simulink subsystem "Rocket_Motor"  (R2020b)
settings: Solver=VariableStepAuto  StartTime=0.0  StopTime=10.0  RelTol=1e-3
libraries: fl_lib x15, nesl_utility x8
settings Model: Creator=Edward  LastModifiedBy=Edward

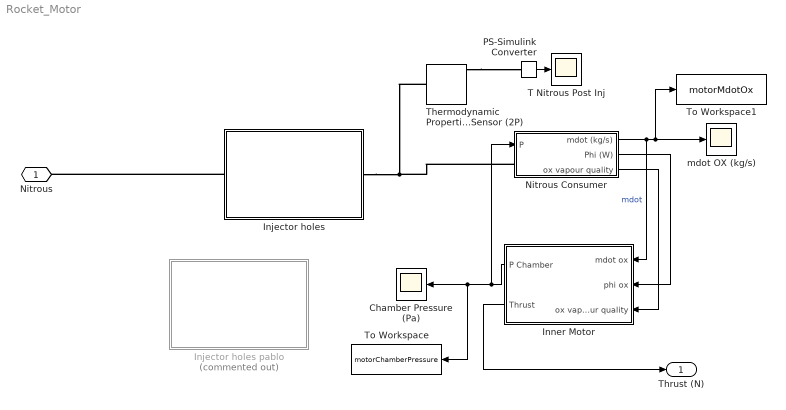
== system Rocket_Motor ==
  Chamber Pressure (Pa) : Scope
  Injector holes : Subsystem  ReferencedSubsystem=Injector
  Injector holes pablo : Subsystem  Commented=on
  Inner Motor : Subsystem
      mask Display: image('$imagefile'); % Use "Edit Image" on toolstrip to change.
  Nitrous Consumer : Subsystem
  PS-Simulink Converter : nesl_utility/PS-Simulink Converter  PhysicalDomain=network_engine_domain  SubClassName=ps_output  LeftPortType=input  RightPortType=output  PseudoPeriodic=off  Frequencies=[]  Unit=inherit  AffineConversion=off
  T Nitrous Post Inj : Scope
  Thermodynamic Properties Sensor (2P) : fl_lib/Two-Phase Fluid/Sensors/Thermodynamic Properties Sensor (2P)
      settings: SourceProductBaseCode=SS  InternalSimscapePortConfiguration="{\"Bottom\":[],\"Left\":[{\"id\":\"A\",\"label\":\"A\",\"type\":\"foundation.two_phase_fluid.two_phase_fluid\"}],\"Right\":[{\"id\":\"T\",\"label\":\"T\",\"type\":\"output\"},{\"id\":\"H\",\"label\":\"h\",\"type\":\"output\"},{\"id\":\"V\",\"label\":\"v\",\"type\":\"output\"},{\"id\":\"S\",\"label\":\"s\",\"type\":\"output\"}],\"Top\":[]}"
  To Workspace : ToWorkspace  VariableName=motorChamberPressure  SaveFormat=Timeseries  SampleTime=-1
  To Workspace1 : ToWorkspace  VariableName=motorMdotOx  SaveFormat=Timeseries  SampleTime=-1
  mdot OX (kg/s) : Scope
  Nitrous : PMIOPort  Side=Left
  Thrust (N) : Outport
  wires:
  Nitrous Consumer/1(mdot (kg/s)) -> mdot OX (kg/s)/1, To Workspace1/1, Inner Motor/1(mdot ox)  "mdot"
  Inner Motor/1(P Chamber) -> To Workspace/1, Chamber Pressure (Pa)/1, Nitrous Consumer/1(P)
  Nitrous Consumer/2(Phi (W)) -> Inner Motor/2(phi ox)
  Inner Motor/2(Thrust) -> Thrust (N)/1
  Nitrous Consumer/3(ox vapour quality) -> Inner Motor/3(ox vapour quality)
  PS-Simulink Converter/1 -> T Nitrous Post Inj/1
  connections:
  Nitrous Consumer/LConn1 -- Thermodynamic Properties Sensor (2P)/LConn1 -- Injector holes/RConn1
  Injector holes/LConn1 -- Nitrous/RConn1
  Thermodynamic Properties Sensor (2P)/RConn1 -- PS-Simulink Converter/LConn1

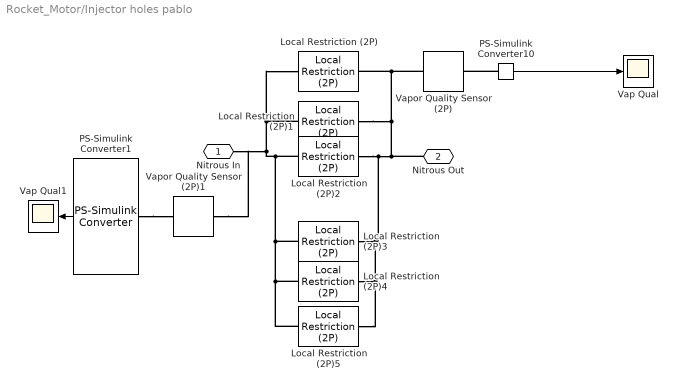
== system Rocket_Motor/Injector holes pablo ==
  Local Restriction (2P) : fl_lib/Two-Phase Fluid/Elements/Local Restriction (2P)  restriction_area=9.50e-7 m^2  area=sim.preInjectorPipe.crossSection m^2  Cd=0.64  B_lam=0.999
      settings: SourceProductBaseCode=SS  InternalSimscapePortConfiguration="{\"Bottom\":[],\"Left\":[{\"id\":\"A\",\"label\":\"A\",\"type\":\"foundation.two_phase_fluid.two_phase_fluid\"}],\"Right\":[{\"id\":\"B\",\"label\":\"B\",\"type\":\"foundation.two_phase_fluid.two_phase_fluid\"}],\"Top\":[]}"
  Local Restriction (2P)1 : fl_lib/Two-Phase Fluid/Elements/Local Restriction (2P)  restriction_area=9.50e-7 m^2  area=sim.preInjectorPipe.crossSection m^2  Cd=0.64  B_lam=0.999
      settings: SourceProductBaseCode=SS  InternalSimscapePortConfiguration="{\"Bottom\":[],\"Left\":[{\"id\":\"A\",\"label\":\"A\",\"type\":\"foundation.two_phase_fluid.two_phase_fluid\"}],\"Right\":[{\"id\":\"B\",\"label\":\"B\",\"type\":\"foundation.two_phase_fluid.two_phase_fluid\"}],\"Top\":[]}"
  Local Restriction (2P)2 : fl_lib/Two-Phase Fluid/Elements/Local Restriction (2P)  restriction_area=9.50e-7 m^2  area=sim.preInjectorPipe.crossSection m^2  Cd=0.64  B_lam=0.999
      settings: SourceProductBaseCode=SS  InternalSimscapePortConfiguration="{\"Bottom\":[],\"Left\":[{\"id\":\"A\",\"label\":\"A\",\"type\":\"foundation.two_phase_fluid.two_phase_fluid\"}],\"Right\":[{\"id\":\"B\",\"label\":\"B\",\"type\":\"foundation.two_phase_fluid.two_phase_fluid\"}],\"Top\":[]}"
  Local Restriction (2P)3 : fl_lib/Two-Phase Fluid/Elements/Local Restriction (2P)  restriction_area=4.07e-7 m^2  area=sim.preInjectorPipe.crossSection m^2  Cd=0.64  B_lam=0.999
      settings: SourceProductBaseCode=SS  InternalSimscapePortConfiguration="{\"Bottom\":[],\"Left\":[{\"id\":\"A\",\"label\":\"A\",\"type\":\"foundation.two_phase_fluid.two_phase_fluid\"}],\"Right\":[{\"id\":\"B\",\"label\":\"B\",\"type\":\"foundation.two_phase_fluid.two_phase_fluid\"}],\"Top\":[]}"
  Local Restriction (2P)4 : fl_lib/Two-Phase Fluid/Elements/Local Restriction (2P)  restriction_area=4.07e-7 m^2  area=sim.preInjectorPipe.crossSection m^2  Cd=0.64  B_lam=0.999
      settings: SourceProductBaseCode=SS  InternalSimscapePortConfiguration="{\"Bottom\":[],\"Left\":[{\"id\":\"A\",\"label\":\"A\",\"type\":\"foundation.two_phase_fluid.two_phase_fluid\"}],\"Right\":[{\"id\":\"B\",\"label\":\"B\",\"type\":\"foundation.two_phase_fluid.two_phase_fluid\"}],\"Top\":[]}"
  Local Restriction (2P)5 : fl_lib/Two-Phase Fluid/Elements/Local Restriction (2P)  restriction_area=4.07e-7 m^2  area=sim.preInjectorPipe.crossSection m^2  Cd=0.64  B_lam=0.999
      settings: SourceProductBaseCode=SS  InternalSimscapePortConfiguration="{\"Bottom\":[],\"Left\":[{\"id\":\"A\",\"label\":\"A\",\"type\":\"foundation.two_phase_fluid.two_phase_fluid\"}],\"Right\":[{\"id\":\"B\",\"label\":\"B\",\"type\":\"foundation.two_phase_fluid.two_phase_fluid\"}],\"Top\":[]}"
  PS-Simulink Converter1 : nesl_utility/PS-Simulink Converter  PhysicalDomain=network_engine_domain  SubClassName=ps_output  LeftPortType=input  RightPortType=output  PseudoPeriodic=off  Frequencies=[]  Unit=inherit  AffineConversion=off
  PS-Simulink Converter10 : nesl_utility/PS-Simulink Converter  PhysicalDomain=network_engine_domain  SubClassName=ps_output  LeftPortType=input  RightPortType=output  PseudoPeriodic=off  Frequencies=[]  Unit=inherit  AffineConversion=off
  Vap Qual : Scope
  Vap Qual1 : Scope
  Vapor Quality Sensor (2P) : fl_lib/Two-Phase Fluid/Sensors/Vapor Quality Sensor (2P)  vapor_fraction_spec=foundation.enum.vapor_fraction_spec.quality
      settings: SourceProductBaseCode=SS  InternalSimscapePortConfiguration="{\"Bottom\":[],\"Left\":[{\"id\":\"A\",\"label\":\"A\",\"type\":\"foundation.two_phase_fluid.two_phase_fluid\"}],\"Right\":[{\"id\":\"X\",\"label\":\"X\",\"type\":\"output\"}],\"Top\":[]}"
  Vapor Quality Sensor (2P)1 : fl_lib/Two-Phase Fluid/Sensors/Vapor Quality Sensor (2P)  vapor_fraction_spec=foundation.enum.vapor_fraction_spec.quality
      settings: SourceProductBaseCode=SS  InternalSimscapePortConfiguration="{\"Bottom\":[],\"Left\":[{\"id\":\"A\",\"label\":\"A\",\"type\":\"foundation.two_phase_fluid.two_phase_fluid\"}],\"Right\":[{\"id\":\"X\",\"label\":\"X\",\"type\":\"output\"}],\"Top\":[]}"
  Nitrous In : PMIOPort  Side=Left
  Nitrous Out : PMIOPort  Port=2  Side=Right
  wires:
  PS-Simulink Converter1/1 -> Vap Qual1/1
  PS-Simulink Converter10/1 -> Vap Qual/1
  connections:
  PS-Simulink Converter1/LConn1 -- Vapor Quality Sensor (2P)1/RConn1
  PS-Simulink Converter10/LConn1 -- Vapor Quality Sensor (2P)/RConn1
  Local Restriction (2P)4/LConn1 -- Local Restriction (2P)5/LConn1 -- Local Restriction (2P)3/LConn1 -- Local Restriction (2P)2/LConn1 -- Vapor Quality Sensor (2P)1/LConn1 -- Nitrous In/RConn1 -- Local Restriction (2P)/LConn1 -- Local Restriction (2P)1/LConn1
  Local Restriction (2P)5/RConn1 -- Local Restriction (2P)4/RConn1 -- Local Restriction (2P)3/RConn1 -- Local Restriction (2P)2/RConn1 -- Local Restriction (2P)/RConn1 -- Vapor Quality Sensor (2P)/LConn1 -- Local Restriction (2P)1/RConn1 -- Nitrous Out/RConn1

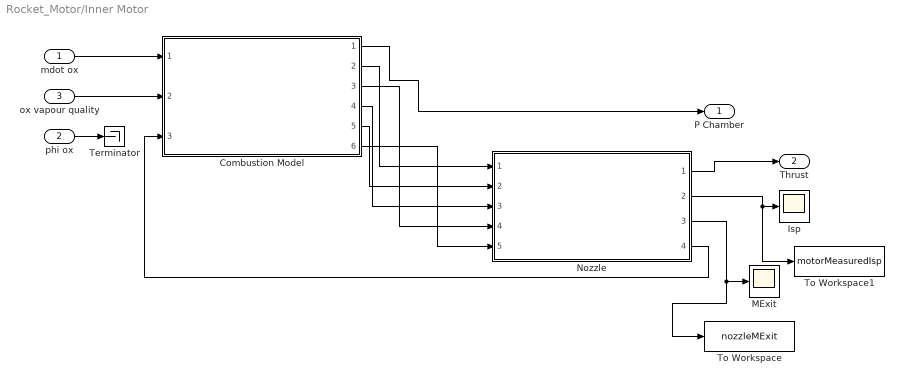
== system Rocket_Motor/Inner Motor ==
  mdot ox : Inport
  phi ox : Inport  Port=2
  ox vapour quality : Inport  Port=3
  Combustion Model : Subsystem  ReferencedSubsystem=Combustion_Model
  Isp : Scope
  MExit : Scope
  Nozzle : Subsystem  ReferencedSubsystem=Nozzle
  Terminator : Terminator
  To Workspace : ToWorkspace  VariableName=nozzleMExit  SaveFormat=Timeseries  SampleTime=-1
  To Workspace1 : ToWorkspace  VariableName=motorMeasuredIsp  SaveFormat=Timeseries  SampleTime=-1
  P Chamber : Outport
  Thrust : Outport  Port=2
  wires:
  Combustion Model/6 -> Nozzle/5
  Nozzle/4 -> Combustion Model/3
  ox vapour quality/1 -> Combustion Model/2
  Combustion Model/3 -> Nozzle/4
  phi ox/1 -> Terminator/1
  Nozzle/3 -> MExit/1, To Workspace/1
  Nozzle/2 -> Isp/1, To Workspace1/1
  Nozzle/1 -> Thrust/1
  Combustion Model/4 -> Nozzle/3
  Combustion Model/5 -> Nozzle/2
  Combustion Model/2 -> Nozzle/1
  Combustion Model/1 -> P Chamber/1
  mdot ox/1 -> Combustion Model/1

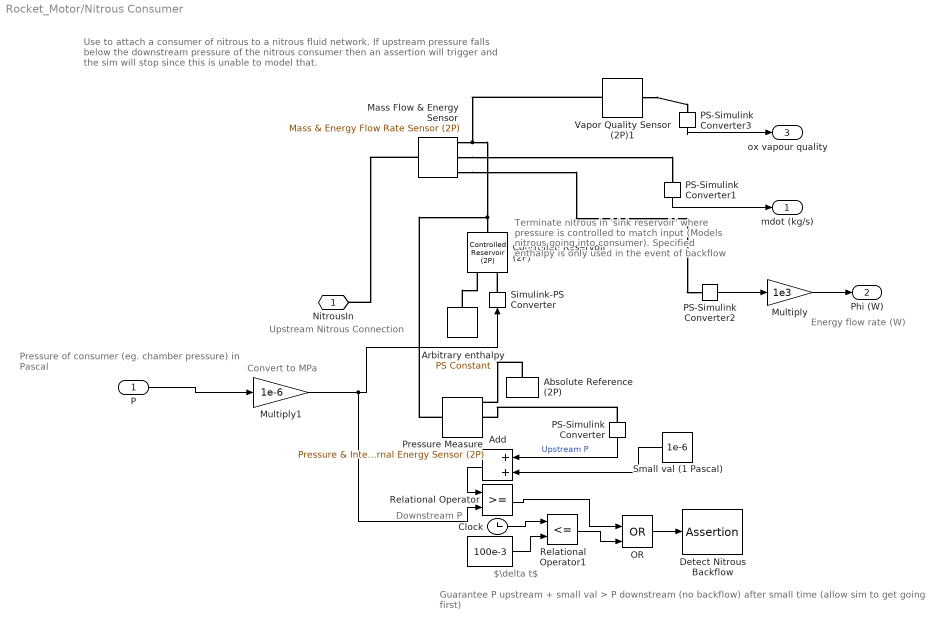
== system Rocket_Motor/Nitrous Consumer ==
  note: Pressure of consumer (eg. chamber pressure)
      | in Pascal
  note: Upstream Nitrous Connection
  note: Energy flow rate (W)
  note: Downstream P
  note: Guarantee P upstream + small val > P downstream (no backflow) after small time (allow sim to get going first)
  note: Terminate nitrous in 'sink reservoir'
      | where pressure is controlled to
      | match input (Models nitrous going into
      | consumer). Specified enthalpy is only used
      | in the event of backflow
  note: Convert to MPa
  note: Use to attach a consumer of nitrous to a nitrous fluid network.
      |
      | If upstream pressure falls below the downstream pressure of the nitrous
      | consumer then an assertion will trigger and the sim will stop since
      | this is unable to model that.
  note: $\delta t$
  P : Inport
  " " : Constant  Value=100e-3
  Absolute Reference (2P) : fl_lib/Two-Phase Fluid/Elements/Absolute Reference (2P)
      settings: SourceProductBaseCode=SS
  Add : Sum
  Arbitrary enthalpy : fl_lib/Physical Signals/Sources/PS Constant  constant=362 kJ/kg
  Clock : Clock
  Controlled Reservoir (2P) : fl_lib/Two-Phase Fluid/Elements/Controlled Reservoir (2P)  energy_spec=foundation.enum.enthalpy_internal_energy_spec.enthalpy  area_A=sim.injector.postInjectorCrossSection m^2
      settings: SourceProductBaseCode=SS  InternalSimscapePortConfiguration="{\"Bottom\":[],\"Left\":[{\"id\":\"A\",\"label\":\"A\",\"type\":\"foundation.two_phase_fluid.two_phase_fluid\"}],\"Right\":[{\"id\":\"H\",\"label\":\"H\",\"type\":\"input\"},{\"id\":\"P\",\"label\":\"P\",\"type\":\"input\"}],\"Top\":[]}"
  Detect Nitrous Backflow : Assertion
  Mass Flow & Energy Sensor : fl_lib/Two-Phase Fluid/Sensors/Mass & Energy Flow Rate Sensor (2P)
      settings: SourceProductBaseCode=SS  InternalSimscapePortConfiguration="{\"Bottom\":[],\"Left\":[{\"id\":\"A\",\"label\":\"A\",\"type\":\"foundation.two_phase_fluid.two_phase_fluid\"}],\"Right\":[{\"id\":\"B\",\"label\":\"B\",\"type\":\"foundation.two_phase_fluid.two_phase_fluid\"},{\"id\":\"M\",\"label\":\"M\",\"type\":\"output\"},{\"id\":\"PHI\",\"label\":\"Phi\",\"type\":\"output\"}],\"Top\":[]}"
  Multiply : Gain  Gain=1e3
  Multiply1 : Gain  Gain=1e-6
  OR : Logic  Operator=OR  IconShape=distinctive  AllPortsSameDT=off  OutDataTypeStr=boolean
  PS-Simulink Converter{,1..3} (4 alike) : nesl_utility/PS-Simulink Converter  PhysicalDomain=network_engine_domain  SubClassName=ps_output  LeftPortType=input  RightPortType=output  PseudoPeriodic=off  Frequencies=[]  Unit=inherit  AffineConversion=off
  Pressure Measure : fl_lib/Two-Phase Fluid/Sensors/Pressure & Internal Energy Sensor (2P)
      settings: SourceProductBaseCode=SS  InternalSimscapePortConfiguration="{\"Bottom\":[],\"Left\":[{\"id\":\"A\",\"label\":\"A\",\"type\":\"foundation.two_phase_fluid.two_phase_fluid\"}],\"Right\":[{\"id\":\"B\",\"label\":\"B\",\"type\":\"foundation.two_phase_fluid.two_phase_fluid\"},{\"id\":\"P\",\"label\":\"P\",\"type\":\"output\"},{\"id\":\"U\",\"label\":\"U\",\"type\":\"output\"}],\"Top\":[]}"
  Relational Operator : RelationalOperator  OutDataTypeStr=boolean  RndMeth=Simplest
  Relational Operator1 : RelationalOperator  Operator=<=  OutDataTypeStr=boolean  RndMeth=Simplest
  Simulink-PS Converter : nesl_utility/Simulink-PS Converter  PhysicalDomain=network_engine_domain  SubClassName=ps_input  LeftPortType=input  RightPortType=output  PseudoPeriodic=off  Frequencies=[]  NoiseDistribution=none  NoiseParameters=[]  Unit=1  AffineConversion=off  FilteringAndDerivatives=provide  SimscapeFilterOrder=1  InputFilterTimeConstant=0.001  UdotUserProvided=0
  Small val (1 Pascal) : Constant  Value=1e-6
  Vapor Quality Sensor (2P)1 : fl_lib/Two-Phase Fluid/Sensors/Vapor Quality Sensor (2P)  vapor_fraction_spec=foundation.enum.vapor_fraction_spec.quality
      settings: SourceProductBaseCode=SS  InternalSimscapePortConfiguration="{\"Bottom\":[],\"Left\":[{\"id\":\"A\",\"label\":\"A\",\"type\":\"foundation.two_phase_fluid.two_phase_fluid\"}],\"Right\":[{\"id\":\"X\",\"label\":\"X\",\"type\":\"output\"}],\"Top\":[]}"
  NitrousIn : PMIOPort  Side=Left
  mdot (kg/s) : Outport
  Phi (W) : Outport  Port=2
  ox vapour quality : Outport  Port=3
  wires:
  OR/1 -> Detect Nitrous Backflow/1
  Relational Operator1/1 -> OR/2
  " "/1 -> Relational Operator1/2
  Clock/1 -> Relational Operator1/1
  Small val (1 Pascal)/1 -> Add/2
  Add/1 -> Relational Operator/1
  PS-Simulink Converter/1 -> Add/1  "Upstream P"
  PS-Simulink Converter3/1 -> ox vapour quality/1
  Multiply1/1 -> Simulink-PS Converter/1, Relational Operator/2
  Multiply/1 -> Phi (W)/1
  PS-Simulink Converter2/1 -> Multiply/1
  P/1 -> Multiply1/1
  PS-Simulink Converter1/1 -> mdot (kg/s)/1
  Relational Operator/1 -> OR/1
  connections:
  Vapor Quality Sensor (2P)1/RConn1 -- PS-Simulink Converter3/LConn1
  Mass Flow & Energy Sensor/LConn1 -- NitrousIn/RConn1
  Mass Flow & Energy Sensor/RConn3 -- PS-Simulink Converter2/LConn1
  Mass Flow & Energy Sensor/RConn2 -- PS-Simulink Converter1/LConn1
  PS-Simulink Converter/LConn1 -- Pressure Measure/RConn2
  Absolute Reference (2P)/LConn1 -- Pressure Measure/RConn1
  Controlled Reservoir (2P)/LConn1 -- Pressure Measure/LConn1 -- Vapor Quality Sensor (2P)1/LConn1 -- Mass Flow & Energy Sensor/RConn1
  Arbitrary enthalpy/RConn1 -- Controlled Reservoir (2P)/RConn1
  Simulink-PS Converter/RConn1 -- Controlled Reservoir (2P)/RConn2
